simulink model "chap17_01_05_mdl"  (R2013b)
settings: Solver=FixedStepDiscrete  StartTime=0.0  StopTime=100  FixedStep=0.01  RelTol=1e-3
InitFcn:
  | config = getActiveConfigSet(bdroot(gcs));
  | st = str2double(get_param(config, 'StartTime'));
  | ed = str2double(get_param(config, 'StopTime'));
  | step = str2double(get_param(config, 'FixedStep'));
  | t = linspace(st, ed, (ed - st)/step + 1)';
  | data_in1 = sin(t);
settings Model: Creator=fnst  LastModifiedBy=sunzx.fnst
settings DataIOCC: ExternalInput=[t, data_in1]
settings OptimizationCC: InlineParams=on  OptimizeModelRefInitCode=on  LifeSpan=1
settings DebuggingCC: InheritedTsInSrcMsg=none
settings HardwareCC: ProdLargestAtomicInteger=Integer  ProdLargestAtomicFloat=Float  ProdIntDivRoundTo=Zero  ProdEndianess=LittleEndian  ProdHWDeviceType=SPANSION Microcontroller->ARM Cortex-M4
settings RTWCC: SystemTargetFile=FM4_PIL.tlc  TemplateMakefile=FM4_PIL.tmf  Description=System Target File for PIL Simulation with FM4 TSP  GenerateReport=on  ProcessScript=FM4_PIL_make_rtw_hook  IncludeHyperlinkInReport=on  LaunchReport=on
settings CodeAppCC: IgnoreCustomStorageClasses=off
settings STFCustomTargetCC: ParMdlRefBuildCompliant=on  IncludeMdlTerminateFcn=off  CombineOutputUpdateFcns=on  ERTFirstTimeCompliant=on  ERTCustomFileBanners=on  SupportContinuousTime=off  SupportNonInlinedSFcns=off  MATLABClassNameForMDSCustomization=Simulink.SoftwareTarget.ERTCustomization  GRTInterface=off  SystemTargetFile=FM4_PIL.tlc
settings ERTTargetCC: CodeReplacementLibrary=ANSI_C  CompOptLevelCompliant=off  ConcurrentExecutionCompliant=off  IncludeMdlTerminateFcn=off  ModelStepFunctionPrototypeControlCompliant=off  CPPClassGenCompliant=off  InlinedParameterPlacement=NonHierarchical  ERTSrcFileBannerTemplate=FM4_PIL_code_template.cgt  ERTHdrFileBannerTemplate=FM4_PIL_code_template.cgt  ERTDataSrcFileTemplate=FM4_PIL_code_template.cgt  ERTDataHdrFileTemplate=FM4_PIL_code_template.cgt  ERTCustomFileTemplate=example_file_process.tlc

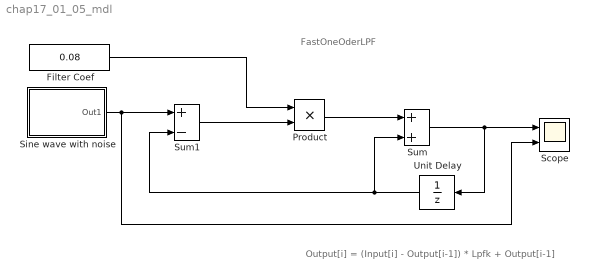
== system chap17_01_05_mdl ==
  note: FastOneOderLPF
  note: Output[i] = (Input[i] - Output[i-1]) * Lpfk + Output[i-1]
  Filter Coef : Constant  Value=0.08
      mask Display: fprintf('Filter coefficient');
  Product : Product  RndMeth=Zero
  Scope : Scope  NumInputPorts=2
      settings: YMin=-5~-5  YMax=5~5
  Sine wave with noise : Subsystem
      mask Display:
      | data = rand(1,150)+ sin([0:0.1:14.9]);
      | plot(data);
  Sum : Sum
  Sum1 : Sum  Inputs=+-
  Unit Delay : UnitDelay  SampleTime=-1
  wires:
  Unit Delay/1 -> Sum/2, Sum1/2
  Product/1 -> Sum/1
  Sum/1 -> Unit Delay/1, Scope/1
  Sine wave with noise/1(Out1) -> Scope/2, Sum1/1
  Sum1/1 -> Product/2
  Filter Coef/1 -> Product/1

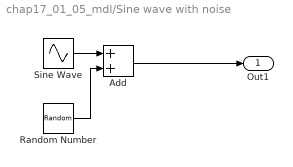
== system chap17_01_05_mdl/Sine wave with noise ==
  Add : Sum
  Random Number : RandomNumber  Variance=0.1
  Sine Wave : Sin  Amplitude=5  Frequency=0.5  SampleTime=0
  Out1 : Outport
  wires:
  Add/1 -> Out1/1
  Random Number/1 -> Add/2
  Sine Wave/1 -> Add/1
